simulink model "MotorControllerAttempt"  (R2021a)
settings: Solver=VariableStepAuto  StartTime=0.0  StopTime=10.0  RelTol=1e-3
values from neighbouring files (symbols this model uses):
  c = cos(theta)    [TorqueMatlabSim.m]
libraries: speedgoatlib_IO691 x8, canmsglib x4, simulink x2, slrealtimeutilitieslib x2
settings Model: Creator=kylec  LastModifiedBy=kylec

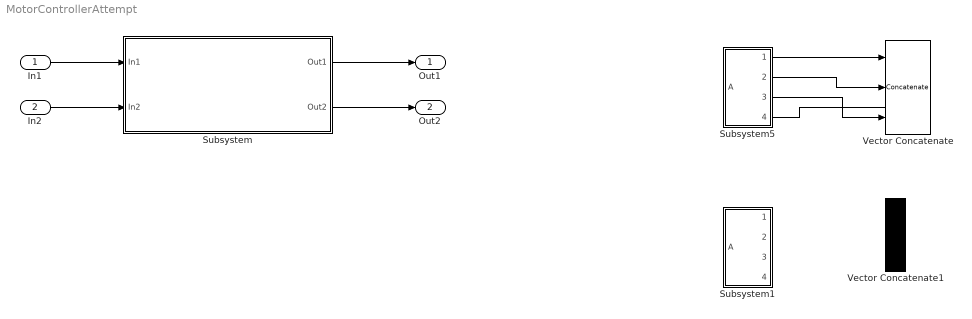
== system MotorControllerAttempt ==
  In1 : Inport
  In2 : Inport  Port=2
  Subsystem : Subsystem
  Subsystem1 : Subsystem
  Subsystem5 : Subsystem
  Vector Concatenate : Concatenate  NumInputs=3
  Vector Concatenate1 : Concatenate
  Out1 : Outport
  Out2 : Outport  Port=2
  wires:
  In1/1 -> Subsystem/1(In1)
  Subsystem/1(Out1) -> Out1/1
  In2/1 -> Subsystem/2(In2)
  Subsystem/2(Out2) -> Out2/1
  Subsystem5/1(Position) -> Vector Concatenate/1
  Subsystem5/2(Velocity) -> Vector Concatenate/2
  Subsystem5/3(Current) -> Vector Concatenate/3
  Subsystem5/4(CAN ID) -> ?

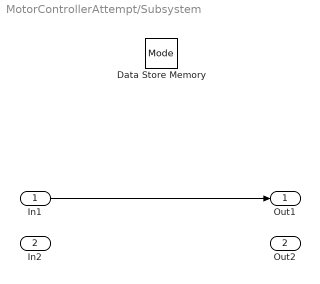
== system MotorControllerAttempt/Subsystem ==
  In1 : Inport
  In2 : Inport  Port=2
  Data Store Memory : DataStoreMemory  DataStoreName=Mode  ReadBeforeWriteMsg=warning  WriteAfterWriteMsg=warning  WriteAfterReadMsg=warning  ShowAdditionalParam=off
  Out1 : Outport
  Out2 : Outport  Port=2
  wires:
  In1/1 -> Out1/1

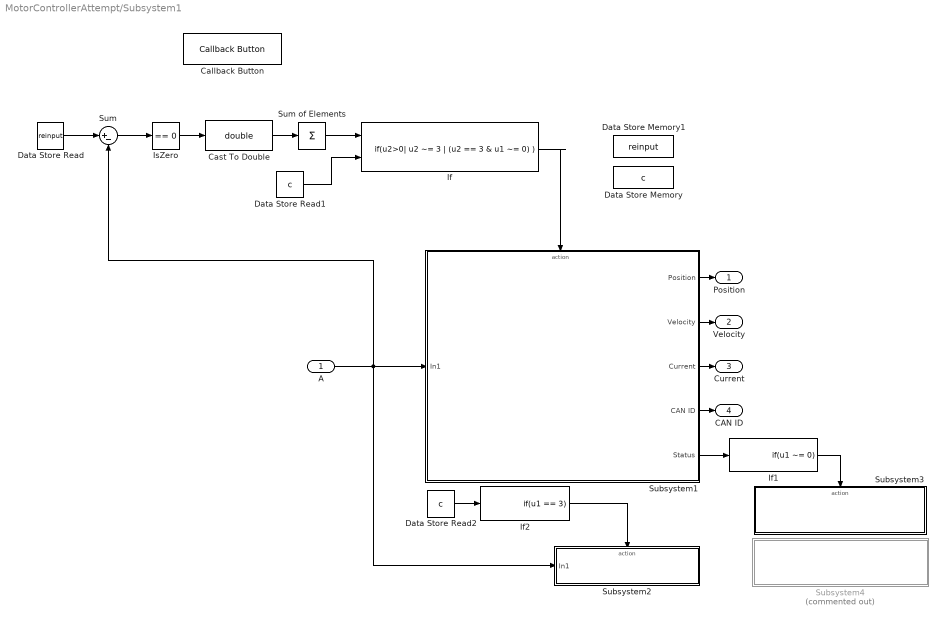
== system MotorControllerAttempt/Subsystem1 ==
  A : Inport
  Callback Button : CallbackButton  StartFcn=c = 0;  ButtonText=deinitiate
      settings: ClickFcn=c = 1;
  Cast To Double : DataTypeConversion  OutDataTypeStr=double
  Data Store Memory : DataStoreMemory  DataStoreName=c  ReadBeforeWriteMsg=warning  WriteAfterWriteMsg=warning  WriteAfterReadMsg=warning  InitialValue=1  ShowAdditionalParam=off  OutMin=1  OutMax=4  OutDataTypeStr=double
  Data Store Memory1 : DataStoreMemory  DataStoreName=reinput  ReadBeforeWriteMsg=warning  WriteAfterWriteMsg=warning  WriteAfterReadMsg=warning  InitialValue=[0,0,0,0,0]  ShowAdditionalParam=off  OutMin=-95.5  OutMax=500  OutDataTypeStr=double
  Data Store Read : DataStoreRead  DataStoreName=reinput  IndexOptions=Index vector (dialog)  Indices=1  OutputSizes=1
  Data Store Read1 : DataStoreRead  DataStoreName=c  IndexOptions=Index vector (dialog)  Indices=1  OutputSizes=1
  Data Store Read2 : DataStoreRead  DataStoreName=c  IndexOptions=Index vector (dialog)  Indices=1  OutputSizes=1
  If : If  NumInputs=2  IfExpression=u2>0| u2 ~= 3 | (u2 == 3 & u1 ~= 0)  ShowElse=off
  If1 : If  IfExpression=u1 ~= 0  ShowElse=off
  If2 : If  IfExpression=u1 == 3  ShowElse=off
  IsZero : simulink/Logic and Bit Operations/Compare To Zero  relop===  OutDataTypeStr=uint8
  Subsystem1 : Subsystem
  Subsystem2 : Subsystem
  Subsystem3 : Subsystem
  Subsystem4 : Subsystem  Commented=on
  Sum : Sum  Inputs=|+-
  Sum of Elements : Sum  Inputs=+  RndMeth=Ceiling
  Position : Outport
  Velocity : Outport  Port=2
  Current : Outport  Port=3
  CAN ID : Outport  Port=4
  wires:
  Data Store Read1/1 -> If/2
  IsZero/1 -> Cast To Double/1
  Subsystem1/5(Status) -> If1/1
  Subsystem1/1(Position) -> Position/1
  A/1 -> Sum/2, Subsystem2/1(In1), Subsystem1/1(In1)
  Data Store Read/1 -> Sum/1
  Data Store Read2/1 -> If2/1
  If2/1 -> Subsystem2/Action
  Cast To Double/1 -> Sum of Elements/1
  If1/1 -> Subsystem3/Action
  Sum/1 -> IsZero/1
  If/1 -> Subsystem1/Action
  Sum of Elements/1 -> If/1
  Subsystem1/3(Current) -> Current/1
  Subsystem1/4(CAN ID) -> CAN ID/1
  Subsystem1/2(Velocity) -> Velocity/1

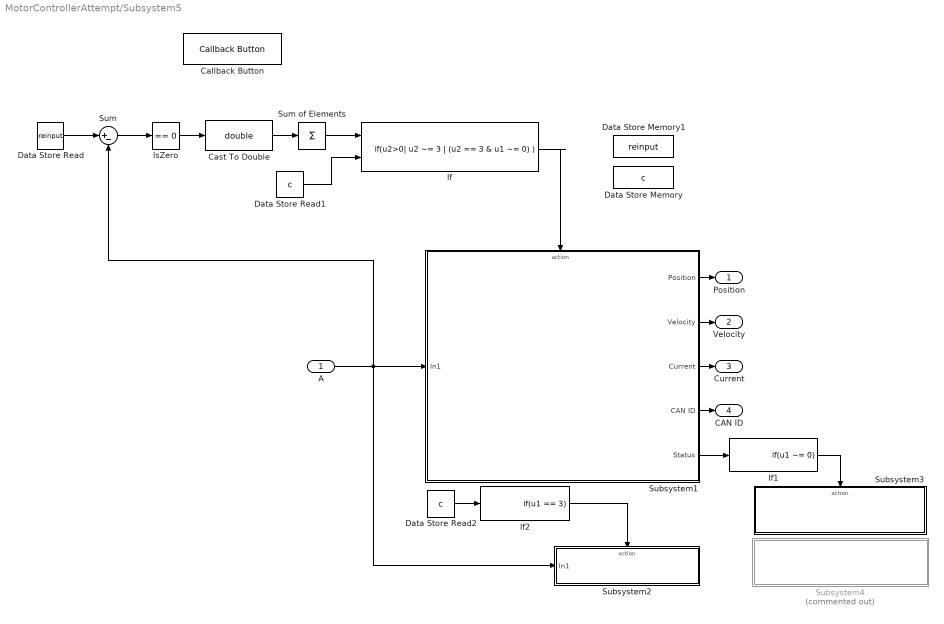
== system MotorControllerAttempt/Subsystem5 ==
  A : Inport
  Callback Button : CallbackButton  StartFcn=c = 0;  ButtonText=deinitiate
      settings: ClickFcn=c = 1;
  Cast To Double : DataTypeConversion  OutDataTypeStr=double
  Data Store Memory : DataStoreMemory  DataStoreName=c  ReadBeforeWriteMsg=warning  WriteAfterWriteMsg=warning  WriteAfterReadMsg=warning  InitialValue=1  ShowAdditionalParam=off  OutMin=1  OutMax=4  OutDataTypeStr=double
  Data Store Memory1 : DataStoreMemory  DataStoreName=reinput  ReadBeforeWriteMsg=warning  WriteAfterWriteMsg=warning  WriteAfterReadMsg=warning  InitialValue=[0,0,0,0,0]  ShowAdditionalParam=off  OutMin=-95.5  OutMax=500  OutDataTypeStr=double
  Data Store Read : DataStoreRead  DataStoreName=reinput  IndexOptions=Index vector (dialog)  Indices=1  OutputSizes=1
  Data Store Read1 : DataStoreRead  DataStoreName=c  IndexOptions=Index vector (dialog)  Indices=1  OutputSizes=1
  Data Store Read2 : DataStoreRead  DataStoreName=c  IndexOptions=Index vector (dialog)  Indices=1  OutputSizes=1
  If : If  NumInputs=2  IfExpression=u2>0| u2 ~= 3 | (u2 == 3 & u1 ~= 0)  ShowElse=off
  If1 : If  IfExpression=u1 ~= 0  ShowElse=off
  If2 : If  IfExpression=u1 == 3  ShowElse=off
  IsZero : simulink/Logic and Bit Operations/Compare To Zero  relop===  OutDataTypeStr=uint8
  Subsystem1 : Subsystem
  Subsystem2 : Subsystem
  Subsystem3 : Subsystem
  Subsystem4 : Subsystem  Commented=on
  Sum : Sum  Inputs=|+-
  Sum of Elements : Sum  Inputs=+  RndMeth=Ceiling
  Position : Outport
  Velocity : Outport  Port=2
  Current : Outport  Port=3
  CAN ID : Outport  Port=4
  wires:
  Data Store Read1/1 -> If/2
  IsZero/1 -> Cast To Double/1
  Subsystem1/5(Status) -> If1/1
  Subsystem1/1(Position) -> Position/1
  A/1 -> Sum/2, Subsystem2/1(In1), Subsystem1/1(In1)
  Data Store Read/1 -> Sum/1
  Data Store Read2/1 -> If2/1
  If2/1 -> Subsystem2/Action
  Cast To Double/1 -> Sum of Elements/1
  If1/1 -> Subsystem3/Action
  Sum/1 -> IsZero/1
  If/1 -> Subsystem1/Action
  Sum of Elements/1 -> If/1
  Subsystem1/3(Current) -> Current/1
  Subsystem1/4(CAN ID) -> CAN ID/1
  Subsystem1/2(Velocity) -> Velocity/1

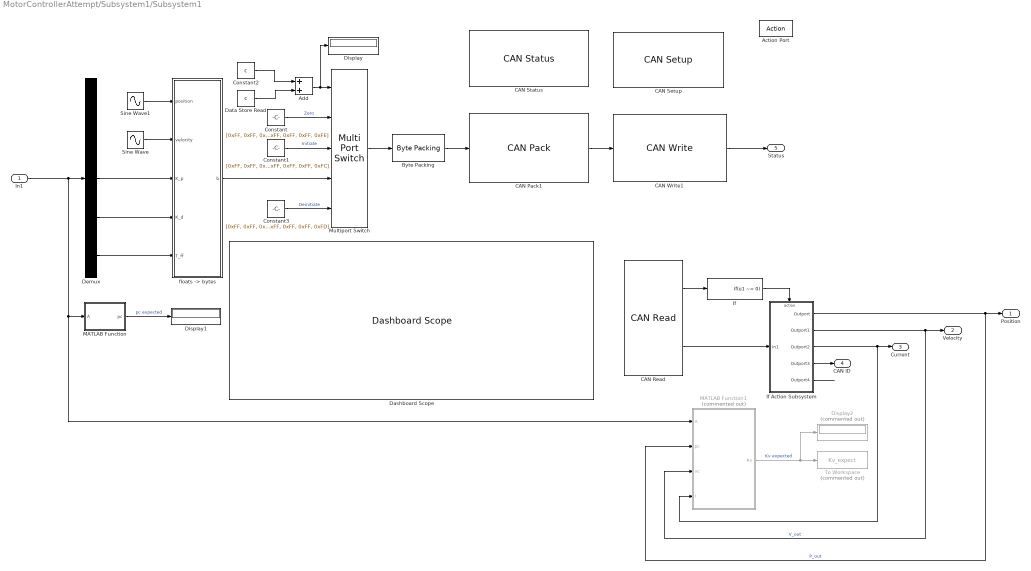
== system MotorControllerAttempt/Subsystem1/Subsystem1 ==
  In1 : Inport
  Action Port : ActionPort
  Add : Sum
  Byte Packing : slrealtimeutilitieslib/Byte Packing  MaskPackedDataType=uint8  MaskUnpackedDataTypes={['uint8']}  MaskAlignment=1
  CAN Pack1 : canmsglib/CAN Pack  MsgList=(none)  MsgName=CAN Msg  MsgIDType=Standard (11-bit identifier)  MsgIdentifier=1  MsgLength=8  Remote=off  ApplyMinMax=off  BusOutput=off  SignalInfo={ 'b1', '0', '8', 'LE', 'unsigned', 'Standard', '0', '1', '0', '-Inf', 'Inf'; 'b2', '8', '8', 'LE', 'unsigned', 'Standard', '0', '1', '0', '-Inf', 'Inf'; 'b3', '16', '8', 'LE', 'unsigned', 'Standard', '0', '1', '0', '-Inf', 'Inf'; 'b4', '24', '8', 'LE', 'unsigned', 'Standard', '0', '1', '0', '-Inf', 'Inf'; 'b5', '32', '8', 'LE', 'unsigned', 'Standard', '0', '1', '0', '-Inf', 'Inf'; 'b6', '40', '8', 'LE', 'unsigned', 'Standard', '0', '1', '0', '-Inf', 'Inf'; 'b7', '48', '8', 'LE', 'unsigned', 'Standard', '0', '1', '0', '-Inf', 'Inf'; 'b8', '56', '8', 'LE', 'unsigned', 'Standard', '0', '1', '0', '-Inf', 'Inf' }
      settings: SourceProductBaseCode=ME,XP,VN  DataFormat=raw data
  CAN Read : speedgoatlib_IO691/CAN Read  id=1  ts=-1  channel=1  messageType=CAN  canType=CAN (HS)  initValues=[691 1 -1 0 1 1]
      settings: SourceProductName=Simulink Real-Time: Speedgoat I/O Blockset
  "CAN Setup " : speedgoatlib_IO691/CAN Setup   moduletype=IO691  id=1  pciSlot=-1  chn1=CAN (HS)  chn2=CAN (HS)  chn3=Disabled  chn4=Disabled  initStruct=[]  termStruct=[]  ArbitrationbdrChn1=1.0 MBaud  ArbitrationManbdrChn1=[2,8,31,8]  FdbdrChn1=5.0 MBaud  FdManbdrChn1=[2,2,5,2]  ArbitrationbdrChn2=1.0 MBaud  ArbitrationManbdrChn2=[2,8,31,8]  FdbdrChn2=5.0 MBaud  FdManbdrChn2=[2,2,5,2]  ArbitrationbdrChn3=1.0 MBaud  ArbitrationManbdrChn3=[2,8,31,8]  FdbdrChn3=5.0 MBaud  FdManbdrChn3=[2,2,5,2]  ArbitrationbdrChn4=1.0 MBaud  ArbitrationManbdrChn4=[2,8,31,8]  FdbdrChn4=5.0 MBaud  FdManbdrChn4=[2,2,5,2]  moduleInitValues=[691 1 -1 -1]
      settings: SourceProductName=Simulink Real-Time: Speedgoat I/O Blockset
  CAN Status : speedgoatlib_IO691/CAN Status  moduleId=1  sampleTime=-1  channel=1  busRecovery=Off  arrayOutput=off  controllerCpuLoad=off  controllerLiveCount=off  initModeAct=off  avgBusLoad=off  receiving=off  RxQueueEmpty=off  dataOverrunRcv=off  rxBufferLevel=off  txPending=off  dataOverrunTx=off  txBufferLevel=off  errWarnLimit=off  errPassLimit=off  errBusOff=off  busRecoveryCounter=off  busCouplingErr=off  transceiverErr=off  opMode=off  brp=off  timeSegment1=off  timeSegment2=off  synchronisationJumpWidth=off  dataTSEG1=off  dataTSEG2=off  dataSJW=off  moduleType=691  qtyStatBlk=1  ptIdx=0  isFDMod=0
      settings: SourceProductName=Simulink Real-Time: Speedgoat I/O Blockset
  CAN Write1 : speedgoatlib_IO691/CAN Write  id=1  ts=-1  channel=1  messageType=CAN  enableStatusPort=on  canType=CAN (HS)  initValues=[691 1 -1 0 1 1 1]
      settings: SourceProductName=Simulink Real-Time: Speedgoat I/O Blockset
  Constant : Constant  Value=[0xFF, 0xFF, 0xFF, 0xFF, 0xFF, 0xFF, 0xFF, 0xFE]
  Constant1 : Constant  Value=[0xFF, 0xFF, 0xFF, 0xFF, 0xFF, 0xFF, 0xFF, 0xFC]
  Constant2 : Constant  Value=c
  Constant3 : Constant  Value=[0xFF, 0xFF, 0xFF, 0xFF, 0xFF, 0xFF, 0xFF, 0xFD]
  Dashboard Scope : DashboardScope
  Data Store Read : DataStoreRead  DataStoreName=c  IndexOptions=Index vector (dialog)  Indices=1  OutputSizes=1
  Demux : Demux  Outputs=5
  Display : Display
  Display1 : Display
  Display2 : Display  Commented=on
  If : If  IfExpression=u1 ~= 0  ShowElse=off
  If Action Subsystem : Subsystem  TreatAsAtomicUnit=on
  MATLAB Function : MATLAB Function  TreatAsAtomicUnit=on
  MATLAB Function1 : MATLAB Function  Commented=on  TreatAsAtomicUnit=on
  Multiport Switch : MultiPortSwitch  Inputs=4
  Sine Wave : Sin  Amplitude=pi/2  Frequency=2*pi/3  Phase=pi/2  SampleTime=0
  Sine Wave1 : Sin  Amplitude=pi/2  Frequency=2*pi/3  SampleTime=0
  To Workspace : ToWorkspace  Commented=on  VariableName=Kv_expect  SaveFormat=Timeseries  SampleTime=-1
  "floats -> bytes" : MATLAB Function  TreatAsAtomicUnit=on
  Position : Outport
  Velocity : Outport  Port=2
  Current : Outport  Port=3
  CAN ID : Outport  Port=4
  Status : Outport  Port=5
  wires:
  Demux/3 -> "floats -> bytes"/3(K_p)
  "floats -> bytes"/1(b) -> Multiport Switch/4
  CAN Read/1 -> If/1
  Demux/5 -> "floats -> bytes"/5(T_ff)
  Constant3/1 -> Multiport Switch/5  "Deinitiate"
  CAN Pack1/1 -> CAN Write1/1
  Constant1/1 -> Multiport Switch/3  "Initiate"
  Demux/4 -> "floats -> bytes"/4(K_d)
  Constant/1 -> Multiport Switch/2  "Zero"
  Byte Packing/1 -> CAN Pack1/1
  CAN Read/2 -> If Action Subsystem/1(In1)
  Multiport Switch/1 -> Byte Packing/1
  If/1 -> If Action Subsystem/Action
  If Action Subsystem/1(Outport) -> MATLAB Function1/2(pc), Position/1  "P_out"
  If Action Subsystem/3(Outport2) -> MATLAB Function1/4(i), Current/1
  If Action Subsystem/4(Outport3) -> CAN ID/1
  In1/1 -> MATLAB Function1/1(A), MATLAB Function/1(A), Demux/1
  If Action Subsystem/2(Outport1) -> Velocity/1, MATLAB Function1/3(vc)  "V_out"
  MATLAB Function/1(pc) -> Display1/1  "pc expected"
  MATLAB Function1/1(Kv) -> Display2/1, To Workspace/1  "Kv expected"
  If Action Subsystem/5(Outport4) -> ?
  CAN Write1/1 -> Status/1
  Sine Wave/1 -> "floats -> bytes"/2(velocity)
  Sine Wave1/1 -> "floats -> bytes"/1(position)
  Data Store Read/1 -> Add/2
  Constant2/1 -> Add/1
  Add/1 -> Display/1, Multiport Switch/1

== system MotorControllerAttempt/Subsystem1/Subsystem2 ==
  In1 : Inport
  Action Port : ActionPort
  Data Store Write : DataStoreWrite  DataStoreName=reinput  IndexOptions=Index vector (dialog)  Indices=1  OutputSizes=1
  wires:
  In1/1 -> Data Store Write/1

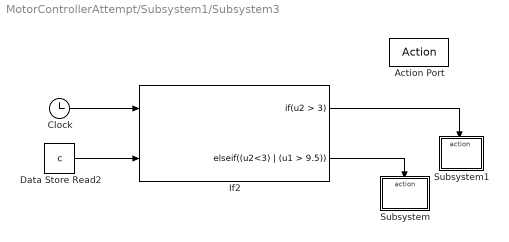
== system MotorControllerAttempt/Subsystem1/Subsystem3 ==
  Action Port : ActionPort
  Clock : Clock
  Data Store Read2 : DataStoreRead  DataStoreName=c  IndexOptions=Index vector (dialog)  Indices=1  OutputSizes=1
  If2 : If  NumInputs=2  IfExpression=u2 > 3  ElseIfExpressions=(u2<3) | (u1 > 9.5)  ShowElse=off
  Subsystem : Subsystem
  Subsystem1 : Subsystem
  wires:
  Clock/1 -> If2/1
  Data Store Read2/1 -> If2/2
  If2/2 -> Subsystem/Action
  If2/1 -> Subsystem1/Action

== system MotorControllerAttempt/Subsystem1/Subsystem4 ==
  Clock : Clock
  If2 : If  IfExpression=(u1 > 19.5)  ShowElse=off
  Subsystem1 : Subsystem
  wires:
  Clock/1 -> If2/1
  If2/1 -> Subsystem1/Action

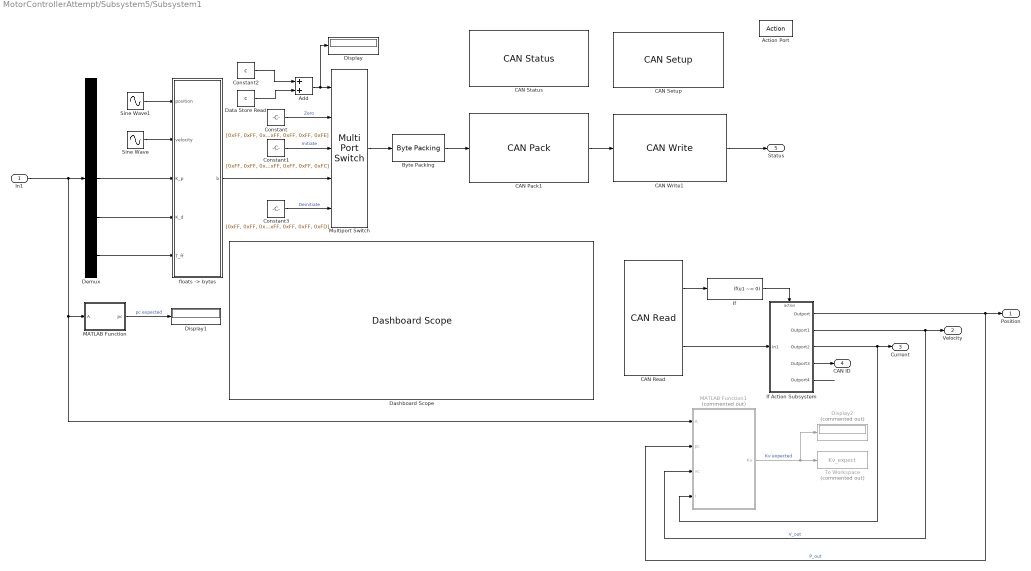
== system MotorControllerAttempt/Subsystem5/Subsystem1 ==
  In1 : Inport
  Action Port : ActionPort  ActionPortLabel=if(u2>0| u2 ~= 3 | (u2 == 3 & u1 ~= 0) )
  Add : Sum
  Byte Packing : slrealtimeutilitieslib/Byte Packing  MaskPackedDataType=uint8  MaskUnpackedDataTypes={['uint8']}  MaskAlignment=1
  CAN Pack1 : canmsglib/CAN Pack  MsgList=(none)  MsgName=CAN Msg  MsgIDType=Standard (11-bit identifier)  MsgIdentifier=1  MsgLength=8  Remote=off  ApplyMinMax=off  BusOutput=off  SignalInfo={ 'b1', '0', '8', 'LE', 'unsigned', 'Standard', '0', '1', '0', '-Inf', 'Inf'; 'b2', '8', '8', 'LE', 'unsigned', 'Standard', '0', '1', '0', '-Inf', 'Inf'; 'b3', '16', '8', 'LE', 'unsigned', 'Standard', '0', '1', '0', '-Inf', 'Inf'; 'b4', '24', '8', 'LE', 'unsigned', 'Standard', '0', '1', '0', '-Inf', 'Inf'; 'b5', '32', '8', 'LE', 'unsigned', 'Standard', '0', '1', '0', '-Inf', 'Inf'; 'b6', '40', '8', 'LE', 'unsigned', 'Standard', '0', '1', '0', '-Inf', 'Inf'; 'b7', '48', '8', 'LE', 'unsigned', 'Standard', '0', '1', '0', '-Inf', 'Inf'; 'b8', '56', '8', 'LE', 'unsigned', 'Standard', '0', '1', '0', '-Inf', 'Inf' }
      settings: SourceProductBaseCode=ME,XP,VN  DataFormat=raw data
  CAN Read : speedgoatlib_IO691/CAN Read  id=1  ts=-1  channel=1  messageType=CAN  canType=CAN (HS)  initValues=[691 1 -1 0 1 1]
      settings: SourceProductName=Simulink Real-Time: Speedgoat I/O Blockset
  "CAN Setup " : speedgoatlib_IO691/CAN Setup   moduletype=IO691  id=1  pciSlot=-1  chn1=CAN (HS)  chn2=CAN (HS)  chn3=Disabled  chn4=Disabled  initStruct=[]  termStruct=[]  ArbitrationbdrChn1=1.0 MBaud  ArbitrationManbdrChn1=[2,8,31,8]  FdbdrChn1=5.0 MBaud  FdManbdrChn1=[2,2,5,2]  ArbitrationbdrChn2=1.0 MBaud  ArbitrationManbdrChn2=[2,8,31,8]  FdbdrChn2=5.0 MBaud  FdManbdrChn2=[2,2,5,2]  ArbitrationbdrChn3=1.0 MBaud  ArbitrationManbdrChn3=[2,8,31,8]  FdbdrChn3=5.0 MBaud  FdManbdrChn3=[2,2,5,2]  ArbitrationbdrChn4=1.0 MBaud  ArbitrationManbdrChn4=[2,8,31,8]  FdbdrChn4=5.0 MBaud  FdManbdrChn4=[2,2,5,2]  moduleInitValues=[691 1 -1 -1]
      settings: SourceProductName=Simulink Real-Time: Speedgoat I/O Blockset
  CAN Status : speedgoatlib_IO691/CAN Status  moduleId=1  sampleTime=-1  channel=1  busRecovery=Off  arrayOutput=off  controllerCpuLoad=off  controllerLiveCount=off  initModeAct=off  avgBusLoad=off  receiving=off  RxQueueEmpty=off  dataOverrunRcv=off  rxBufferLevel=off  txPending=off  dataOverrunTx=off  txBufferLevel=off  errWarnLimit=off  errPassLimit=off  errBusOff=off  busRecoveryCounter=off  busCouplingErr=off  transceiverErr=off  opMode=off  brp=off  timeSegment1=off  timeSegment2=off  synchronisationJumpWidth=off  dataTSEG1=off  dataTSEG2=off  dataSJW=off  moduleType=691  qtyStatBlk=1  ptIdx=0  isFDMod=0
      settings: SourceProductName=Simulink Real-Time: Speedgoat I/O Blockset
  CAN Write1 : speedgoatlib_IO691/CAN Write  id=1  ts=-1  channel=1  messageType=CAN  enableStatusPort=on  canType=CAN (HS)  initValues=[691 1 -1 0 1 1 1]
      settings: SourceProductName=Simulink Real-Time: Speedgoat I/O Blockset
  Constant : Constant  Value=[0xFF, 0xFF, 0xFF, 0xFF, 0xFF, 0xFF, 0xFF, 0xFE]
  Constant1 : Constant  Value=[0xFF, 0xFF, 0xFF, 0xFF, 0xFF, 0xFF, 0xFF, 0xFC]
  Constant2 : Constant  Value=c
  Constant3 : Constant  Value=[0xFF, 0xFF, 0xFF, 0xFF, 0xFF, 0xFF, 0xFF, 0xFD]
  Dashboard Scope : DashboardScope
  Data Store Read : DataStoreRead  DataStoreName=c  IndexOptions=Index vector (dialog)  Indices=1  OutputSizes=1
  Demux : Demux  Outputs=5
  Display : Display
  Display1 : Display
  Display2 : Display  Commented=on
  If : If  IfExpression=u1 ~= 0  ShowElse=off
  If Action Subsystem : Subsystem  TreatAsAtomicUnit=on
  MATLAB Function : MATLAB Function  TreatAsAtomicUnit=on
  MATLAB Function1 : MATLAB Function  Commented=on  TreatAsAtomicUnit=on
  Multiport Switch : MultiPortSwitch  Inputs=4
  Sine Wave : Sin  Amplitude=pi/2  Frequency=2*pi/3  Phase=pi/2  SampleTime=0
  Sine Wave1 : Sin  Amplitude=pi/2  Frequency=2*pi/3  SampleTime=0
  To Workspace : ToWorkspace  Commented=on  VariableName=Kv_expect  SaveFormat=Timeseries  SampleTime=-1
  "floats -> bytes" : MATLAB Function  TreatAsAtomicUnit=on
  Position : Outport
  Velocity : Outport  Port=2
  Current : Outport  Port=3
  CAN ID : Outport  Port=4
  Status : Outport  Port=5
  wires:
  Demux/3 -> "floats -> bytes"/3(K_p)
  "floats -> bytes"/1(b) -> Multiport Switch/4
  CAN Read/1 -> If/1
  Demux/5 -> "floats -> bytes"/5(T_ff)
  Constant3/1 -> Multiport Switch/5  "Deinitiate"
  CAN Pack1/1 -> CAN Write1/1
  Constant1/1 -> Multiport Switch/3  "Initiate"
  Demux/4 -> "floats -> bytes"/4(K_d)
  Constant/1 -> Multiport Switch/2  "Zero"
  Byte Packing/1 -> CAN Pack1/1
  CAN Read/2 -> If Action Subsystem/1(In1)
  Multiport Switch/1 -> Byte Packing/1
  If/1 -> If Action Subsystem/Action
  If Action Subsystem/1(Outport) -> MATLAB Function1/2(pc), Position/1  "P_out"
  If Action Subsystem/3(Outport2) -> MATLAB Function1/4(i), Current/1
  If Action Subsystem/4(Outport3) -> CAN ID/1
  In1/1 -> MATLAB Function1/1(A), MATLAB Function/1(A), Demux/1
  If Action Subsystem/2(Outport1) -> Velocity/1, MATLAB Function1/3(vc)  "V_out"
  MATLAB Function/1(pc) -> Display1/1  "pc expected"
  MATLAB Function1/1(Kv) -> Display2/1, To Workspace/1  "Kv expected"
  If Action Subsystem/5(Outport4) -> ?
  CAN Write1/1 -> Status/1
  Sine Wave/1 -> "floats -> bytes"/2(velocity)
  Sine Wave1/1 -> "floats -> bytes"/1(position)
  Data Store Read/1 -> Add/2
  Constant2/1 -> Add/1
  Add/1 -> Display/1, Multiport Switch/1

== system MotorControllerAttempt/Subsystem5/Subsystem2 ==
  In1 : Inport
  Action Port : ActionPort  ActionPortLabel=if(u1 == 3)
  Data Store Write : DataStoreWrite  DataStoreName=reinput  IndexOptions=Index vector (dialog)  Indices=1  OutputSizes=1
  wires:
  In1/1 -> Data Store Write/1

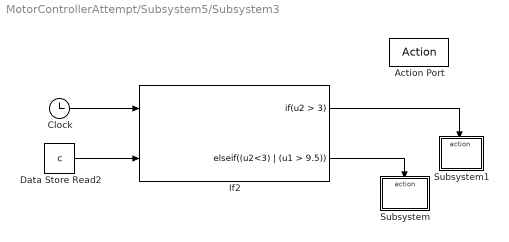
== system MotorControllerAttempt/Subsystem5/Subsystem3 ==
  Action Port : ActionPort  ActionPortLabel=if(u1 ~= 0)
  Clock : Clock
  Data Store Read2 : DataStoreRead  DataStoreName=c  IndexOptions=Index vector (dialog)  Indices=1  OutputSizes=1
  If2 : If  NumInputs=2  IfExpression=u2 > 3  ElseIfExpressions=(u2<3) | (u1 > 9.5)  ShowElse=off
  Subsystem : Subsystem
  Subsystem1 : Subsystem
  wires:
  Clock/1 -> If2/1
  Data Store Read2/1 -> If2/2
  If2/2 -> Subsystem/Action
  If2/1 -> Subsystem1/Action

== system MotorControllerAttempt/Subsystem5/Subsystem4 ==
  Clock : Clock
  If2 : If  IfExpression=(u1 > 19.5)  ShowElse=off
  Subsystem1 : Subsystem
  wires:
  Clock/1 -> If2/1
  If2/1 -> Subsystem1/Action

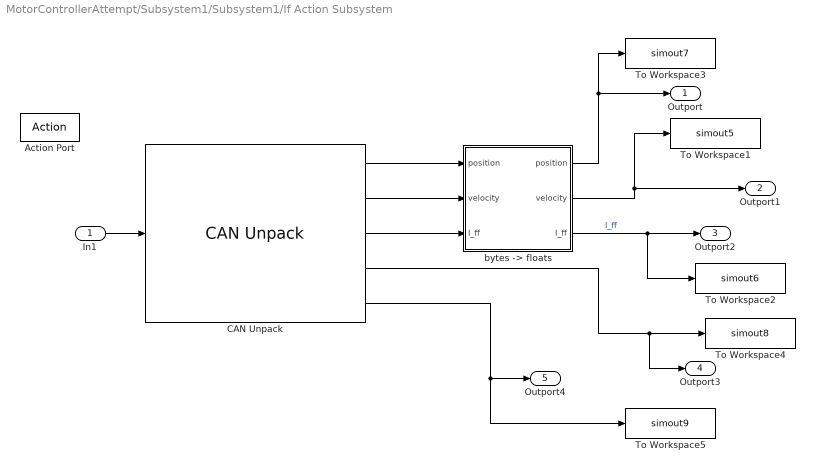
== system MotorControllerAttempt/Subsystem1/Subsystem1/If Action Subsystem ==
  In1 : Inport
  Action Port : ActionPort
  CAN Unpack : canmsglib/CAN Unpack  MsgList=(none)  MsgName=CAN Msg  MsgIDType=Standard (11-bit identifier)  MsgIdentifier=-1  MsgLength=6  SignalInfo={ 'position', '16', '16', 'BE', 'unsigned', 'Standard', '0', '1', '0', '0', '65535'; 'velocity', '36', '12', 'BE', 'unsigned', 'Standard', '0', '1', '0', '0', '4095'; 'current', '40', '12', 'BE', 'unsigned', 'Standard', '0', '1', '0', '0', '4095'; 'id', '0', '8', 'BE', 'unsigned', 'Standard', '0', '1', '0', '0', '255' }  IDPort=off  TimestampPort=off  ErrorPort=off  RemotePort=off  LengthPort=off  StatusPort=on  ApplyMinMax=off
      settings: SourceProductBaseCode=ME,XP,VN
  To Workspace1 : ToWorkspace  VariableName=simout5  SampleTime=-1
  To Workspace2 : ToWorkspace  VariableName=simout6  SampleTime=-1
  To Workspace3 : ToWorkspace  VariableName=simout7  SampleTime=-1
  To Workspace4 : ToWorkspace  VariableName=simout8  SampleTime=-1
  To Workspace5 : ToWorkspace  VariableName=simout9  SampleTime=-1
  "bytes -> floats" : MATLAB Function  TreatAsAtomicUnit=on
  Outport : Outport
  Outport1 : Outport  Port=2
  Outport2 : Outport  Port=3
  Outport3 : Outport  Port=4
  Outport4 : Outport  Port=5
  wires:
  CAN Unpack/5 -> Outport4/1, To Workspace5/1
  CAN Unpack/1 -> "bytes -> floats"/1("position ")
  CAN Unpack/3 -> "bytes -> floats"/3("I_ff ")
  "bytes -> floats"/1(position) -> Outport/1, To Workspace3/1
  CAN Unpack/4 -> Outport3/1, To Workspace4/1
  "bytes -> floats"/2(velocity) -> Outport1/1, To Workspace1/1
  "bytes -> floats"/3(I_ff) -> Outport2/1, To Workspace2/1  "I_ff"
  CAN Unpack/2 -> "bytes -> floats"/2("velocity ")
  In1/1 -> CAN Unpack/1

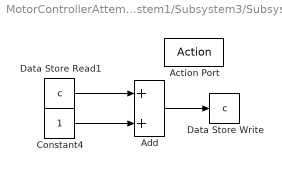
== system MotorControllerAttempt/Subsystem1/Subsystem3/Subsystem ==
  Action Port : ActionPort
  Add : Sum
  Constant4 : Constant
  Data Store Read1 : DataStoreRead  DataStoreName=c  IndexOptions=Index vector (dialog)  Indices=1  OutputSizes=1
  Data Store Write : DataStoreWrite  DataStoreName=c  IndexOptions=Index vector (dialog)  Indices=1  OutputSizes=1
  wires:
  Data Store Read1/1 -> Add/1
  Constant4/1 -> Add/2
  Add/1 -> Data Store Write/1

== system MotorControllerAttempt/Subsystem1/Subsystem3/Subsystem1 ==
  Action Port : ActionPort
  Constant5 : Constant
  Stop Simulation : Stop
  wires:
  Constant5/1 -> Stop Simulation/1

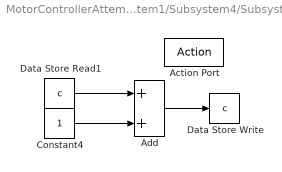
== system MotorControllerAttempt/Subsystem1/Subsystem4/Subsystem1 ==
  Action Port : ActionPort
  Add : Sum
  Constant4 : Constant
  Data Store Read1 : DataStoreRead  DataStoreName=c  IndexOptions=Index vector (dialog)  Indices=1  OutputSizes=1
  Data Store Write : DataStoreWrite  DataStoreName=c  IndexOptions=Index vector (dialog)  Indices=1  OutputSizes=1
  wires:
  Data Store Read1/1 -> Add/1
  Constant4/1 -> Add/2
  Add/1 -> Data Store Write/1

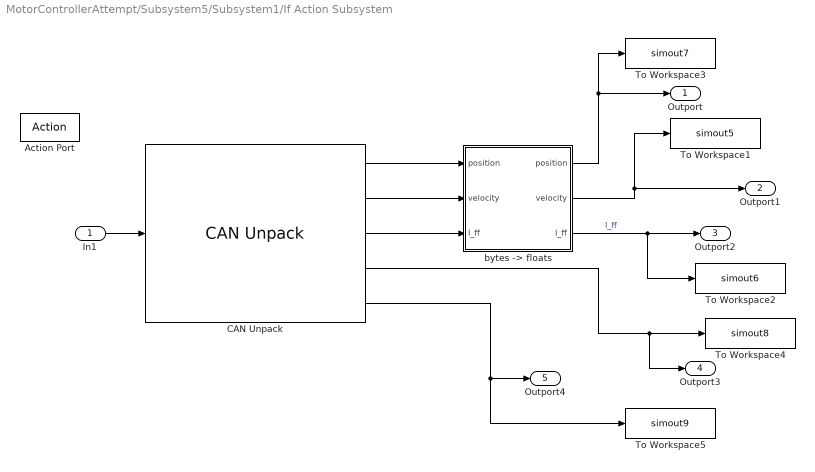
== system MotorControllerAttempt/Subsystem5/Subsystem1/If Action Subsystem ==
  In1 : Inport
  Action Port : ActionPort
  CAN Unpack : canmsglib/CAN Unpack  MsgList=(none)  MsgName=CAN Msg  MsgIDType=Standard (11-bit identifier)  MsgIdentifier=-1  MsgLength=6  SignalInfo={ 'position', '16', '16', 'BE', 'unsigned', 'Standard', '0', '1', '0', '0', '65535'; 'velocity', '36', '12', 'BE', 'unsigned', 'Standard', '0', '1', '0', '0', '4095'; 'current', '40', '12', 'BE', 'unsigned', 'Standard', '0', '1', '0', '0', '4095'; 'id', '0', '8', 'BE', 'unsigned', 'Standard', '0', '1', '0', '0', '255' }  IDPort=off  TimestampPort=off  ErrorPort=off  RemotePort=off  LengthPort=off  StatusPort=on  ApplyMinMax=off
      settings: SourceProductBaseCode=ME,XP,VN
  To Workspace1 : ToWorkspace  VariableName=simout5  SampleTime=-1
  To Workspace2 : ToWorkspace  VariableName=simout6  SampleTime=-1
  To Workspace3 : ToWorkspace  VariableName=simout7  SampleTime=-1
  To Workspace4 : ToWorkspace  VariableName=simout8  SampleTime=-1
  To Workspace5 : ToWorkspace  VariableName=simout9  SampleTime=-1
  "bytes -> floats" : MATLAB Function  TreatAsAtomicUnit=on
  Outport : Outport
  Outport1 : Outport  Port=2
  Outport2 : Outport  Port=3
  Outport3 : Outport  Port=4
  Outport4 : Outport  Port=5
  wires:
  CAN Unpack/5 -> Outport4/1, To Workspace5/1
  CAN Unpack/1 -> "bytes -> floats"/1("position ")
  CAN Unpack/3 -> "bytes -> floats"/3("I_ff ")
  "bytes -> floats"/1(position) -> Outport/1, To Workspace3/1
  CAN Unpack/4 -> Outport3/1, To Workspace4/1
  "bytes -> floats"/2(velocity) -> Outport1/1, To Workspace1/1
  "bytes -> floats"/3(I_ff) -> Outport2/1, To Workspace2/1  "I_ff"
  CAN Unpack/2 -> "bytes -> floats"/2("velocity ")
  In1/1 -> CAN Unpack/1

== system MotorControllerAttempt/Subsystem5/Subsystem3/Subsystem ==
  Action Port : ActionPort
  Add : Sum
  Constant4 : Constant
  Data Store Read1 : DataStoreRead  DataStoreName=c  IndexOptions=Index vector (dialog)  Indices=1  OutputSizes=1
  Data Store Write : DataStoreWrite  DataStoreName=c  IndexOptions=Index vector (dialog)  Indices=1  OutputSizes=1
  wires:
  Data Store Read1/1 -> Add/1
  Constant4/1 -> Add/2
  Add/1 -> Data Store Write/1

== system MotorControllerAttempt/Subsystem5/Subsystem3/Subsystem1 ==
  Action Port : ActionPort
  Constant5 : Constant
  Stop Simulation : Stop
  wires:
  Constant5/1 -> Stop Simulation/1

== system MotorControllerAttempt/Subsystem5/Subsystem4/Subsystem1 ==
  Action Port : ActionPort
  Add : Sum
  Constant4 : Constant
  Data Store Read1 : DataStoreRead  DataStoreName=c  IndexOptions=Index vector (dialog)  Indices=1  OutputSizes=1
  Data Store Write : DataStoreWrite  DataStoreName=c  IndexOptions=Index vector (dialog)  Indices=1  OutputSizes=1
  wires:
  Data Store Read1/1 -> Add/1
  Constant4/1 -> Add/2
  Add/1 -> Data Store Write/1

== matlab function MotorControllerAttempt/Subsystem5/Subsystem1/floats -> bytes ==
  data: position input; b output uint8 size=8; velocity input; K_p input; K_d input; T_ff input
function b = fcn(position, velocity, K_p, K_d, T_ff)

P_MIN  =-95.5;  % [rad]
P_MAX  = 95.5;  % [rad]
V_MIN  =-45;    % [rad/s] 30 to 45
V_MAX  = 45;    % [rad/s]
KP_MIN = 0;     % [Nm/rad]
KP_MAX = 500;   % [Nm/rad]
KD_MIN = 0;     % [Nm*s/rad
KD_MAX = 5;     % [Nm*s/rad
T_MIN  =-18;    % [Nm]
T_MAX  = 18;    % [Nm]

position = floor((max(min(position,P_MAX) ,P_MIN)  - P_MIN )*65535/(P_MAX  - P_MIN));
velocity = floor((max(min(velocity,V_MAX) ,V_MIN)  - V_MIN )*4095 /(V_MAX  - V_MIN));
K_p      = floor((max(min(K_p     ,KP_MAX),KP_MIN) - KP_MIN)*4095 /(KP_MAX - KP_MIN));
K_d      = floor((max(min(K_d     ,V_MAX) ,V_MIN)  - KD_MIN)*4095 /(KD_MAX - KD_MIN));
T_ff     = floor((max(min(T_ff    ,V_MAX) ,V_MIN)  - T_MIN )*4095 /(T_MAX  - T_MIN));

p  = dec2bin(position);
p  = [repmat('0', 1, 16-length(p)),p];
v  = dec2bin(velocity);
v  = [repmat('0', 1, 12-length(v)),v];
kp = dec2bin(K_p);
kp  = [repmat('0', 1, 12-length(kp)),kp];
kd = dec2bin(K_d);
kd  = [repmat('0', 1, 12-length(kd)),kd];
t  = dec2bin(T_ff);
t  = [repmat('0', 1, 12-length(t)),t];

B = repmat('0', 8, 8);

B(1,:) = p(1:8);
B(2,:) = p(9:16);
B(3,:) = v(1:8);
B(4,:) = [v(9:12),kp(1:4)];
B(5,:) = kp(5:12);
B(6,:) = kd(1:8);
B(7,:) = [kd(9:12),t(1:4)];
B(8,:) = t(5:12);

B  = bin2dec(B);

b = uint8(B);

== matlab function MotorControllerAttempt/Subsystem5/Subsystem1/If Action Subsystem/bytes -> floats ==
  data: position input; position output; velocity output; I_ff output; velocity input; I_ff input
function [position, velocity, I_ff] = fcn(position, velocity, I_ff)

P_MIN  =-95.5;  % [rad]
P_MAX  = 95.5;  % [rad]
V_MIN  =-45;    % [rad/s]
V_MAX  = 45;    % [rad/s]
I_MIN  =-40;    % []
I_MAX  = 40;    % []

position = position*(P_MAX  - P_MIN)/65535+ P_MIN;
velocity = velocity*(V_MAX  - V_MIN)/4095 + V_MIN;
I_ff     = I_ff*(I_MAX  - I_MIN)/4095 + I_MIN;

== matlab function MotorControllerAttempt/Subsystem5/Subsystem1/MATLAB Function ==
  data: A input; pc output
function pc  = getPc(A)
    pc = (A(4)*A(2) + A(5))/A(3) + A(1);
end

== matlab function MotorControllerAttempt/Subsystem5/Subsystem1/MATLAB Function1 ==
  data: A input; Kv output; pc input; vc input; i input
function Kv  = getKv(A,pc,vc,i)
    Kv = (A(3)*(A(1)-pc) + A(4)*(A(2) - vc) +A(5))/i;
end

== matlab function MotorControllerAttempt/Subsystem1/Subsystem1/If Action Subsystem/bytes -> floats ==
  data: position input; position output; velocity output; I_ff output; velocity input; I_ff input
function [position, velocity, I_ff] = fcn(position, velocity, I_ff)

P_MIN  =-95.5;  % [rad]
P_MAX  = 95.5;  % [rad]
V_MIN  =-45;    % [rad/s]
V_MAX  = 45;    % [rad/s]
I_MIN  =-40;    % []
I_MAX  = 40;    % []

position = position*(P_MAX  - P_MIN)/65535+ P_MIN;
velocity = velocity*(V_MAX  - V_MIN)/4095 + V_MIN;
I_ff     = I_ff*(I_MAX  - I_MIN)/4095 + I_MIN;

== matlab function MotorControllerAttempt/Subsystem1/Subsystem1/MATLAB Function ==
  data: A input; pc output
function pc  = getPc(A)
    pc = (A(4)*A(2) + A(5))/A(3) + A(1);
end

== matlab function MotorControllerAttempt/Subsystem1/Subsystem1/MATLAB Function1 ==
  data: A input; Kv output; pc input; vc input; i input
function Kv  = getKv(A,pc,vc,i)
    Kv = (A(3)*(A(1)-pc) + A(4)*(A(2) - vc) +A(5))/i;
end

== matlab function MotorControllerAttempt/Subsystem1/Subsystem1/floats -> bytes ==
  data: position input; b output uint8 size=8; velocity input; K_p input; K_d input; T_ff input
function b = fcn(position, velocity, K_p, K_d, T_ff)

P_MIN  =-95.5;  % [rad]
P_MAX  = 95.5;  % [rad]
V_MIN  =-45;    % [rad/s] 30 to 45
V_MAX  = 45;    % [rad/s]
KP_MIN = 0;     % [Nm/rad]
KP_MAX = 500;   % [Nm/rad]
KD_MIN = 0;     % [Nm*s/rad
KD_MAX = 5;     % [Nm*s/rad
T_MIN  =-18;    % [Nm]
T_MAX  = 18;    % [Nm]

position = floor((max(min(position,P_MAX) ,P_MIN)  - P_MIN )*65535/(P_MAX  - P_MIN));
velocity = floor((max(min(velocity,V_MAX) ,V_MIN)  - V_MIN )*4095 /(V_MAX  - V_MIN));
K_p      = floor((max(min(K_p     ,KP_MAX),KP_MIN) - KP_MIN)*4095 /(KP_MAX - KP_MIN));
K_d      = floor((max(min(K_d     ,V_MAX) ,V_MIN)  - KD_MIN)*4095 /(KD_MAX - KD_MIN));
T_ff     = floor((max(min(T_ff    ,V_MAX) ,V_MIN)  - T_MIN )*4095 /(T_MAX  - T_MIN));

p  = dec2bin(position);
p  = [repmat('0', 1, 16-length(p)),p];
v  = dec2bin(velocity);
v  = [repmat('0', 1, 12-length(v)),v];
kp = dec2bin(K_p);
kp  = [repmat('0', 1, 12-length(kp)),kp];
kd = dec2bin(K_d);
kd  = [repmat('0', 1, 12-length(kd)),kd];
t  = dec2bin(T_ff);
t  = [repmat('0', 1, 12-length(t)),t];

B = repmat('0', 8, 8);

B(1,:) = p(1:8);
B(2,:) = p(9:16);
B(3,:) = v(1:8);
B(4,:) = [v(9:12),kp(1:4)];
B(5,:) = kp(5:12);
B(6,:) = kd(1:8);
B(7,:) = [kd(9:12),t(1:4)];
B(8,:) = t(5:12);

B  = bin2dec(B);

b = uint8(B);
